simulink model "untitled1"  (R2022a)
settings: Solver=FixedStepDiscrete  StartTime=0.0  StopTime=0.2  FixedStep=0.001  RelTol=1e-3
settings Model: Creator=Administrator  LastModifiedBy=Administrator

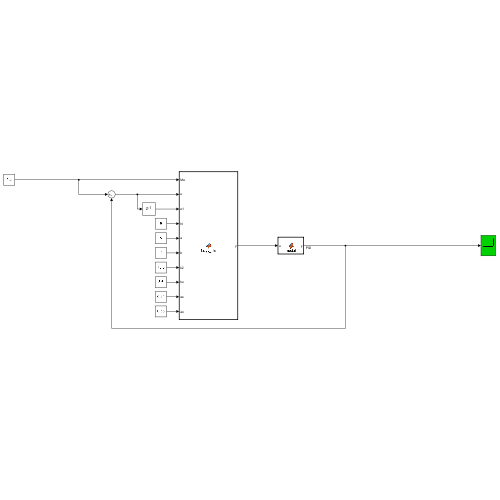
[thumbnail: Simulink's stored preview of the top-level diagram]
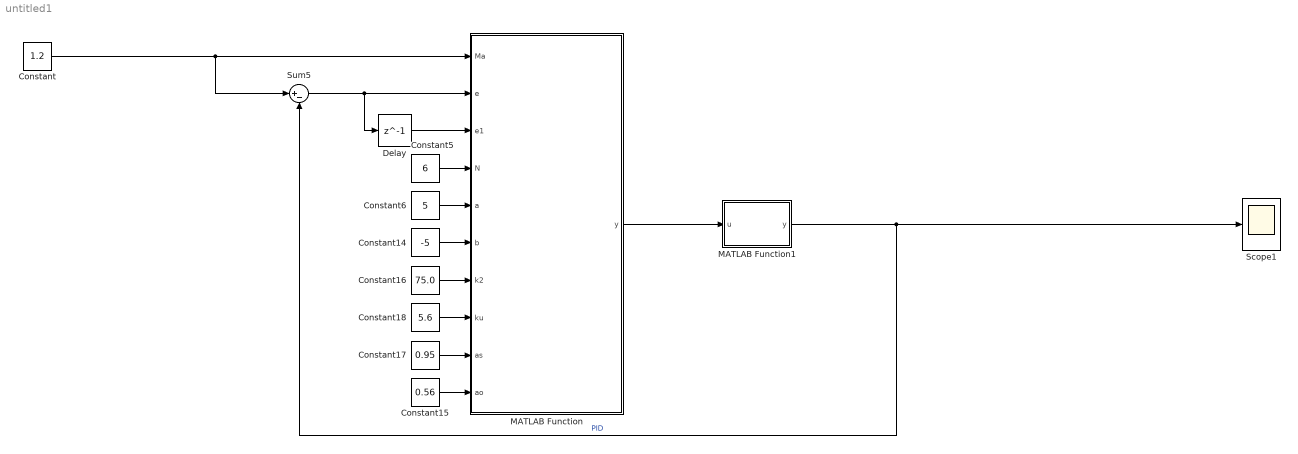
== system untitled1 ==
  Constant : Constant  Value=1.2
  Constant14 : Constant  Value=-5  OutDataTypeStr=Inherit: Inherit via back propagation
  Constant15 : Constant  Value=0.56  OutDataTypeStr=Inherit: Inherit via back propagation
  Constant16 : Constant  Value=75.0  OutDataTypeStr=Inherit: Inherit via back propagation
  Constant17 : Constant  Value=0.95  OutDataTypeStr=Inherit: Inherit via back propagation
  Constant18 : Constant  Value=5.6  OutDataTypeStr=Inherit: Inherit via back propagation
  Constant5 : Constant  Value=6  OutDataTypeStr=Inherit: Inherit via back propagation
  Constant6 : Constant  Value=5
  Delay : Delay  DelayLength=1
  MATLAB Function : MATLAB Function  TreatAsAtomicUnit=on
      settings: MinAlgLoopOccurrences=on
  MATLAB Function1 : MATLAB Function  TreatAsAtomicUnit=on
  Scope1 : Scope
  Sum5 : Sum  Inputs=|+-
  wires:
  Constant6/1 -> MATLAB Function/5(a)
  Constant18/1 -> MATLAB Function/8(ku)
  Constant15/1 -> MATLAB Function/10(ao)
  Sum5/1 -> Delay/1, MATLAB Function/2(e)
  Constant5/1 -> MATLAB Function/4(N)
  Constant14/1 -> MATLAB Function/6(b)
  Constant16/1 -> MATLAB Function/7(k2)
  Constant17/1 -> MATLAB Function/9(as)
  Constant/1 -> MATLAB Function/1(Ma), Sum5/1
  Delay/1 -> MATLAB Function/3(e1)
  MATLAB Function1/1(y) -> Sum5/2, Scope1/1  "PID"
  MATLAB Function/1(y) -> MATLAB Function1/1(u)

== matlab function untitled1/MATLAB Function1 ==
  data: u input; y output
function y = model(u)

y1 = (50)/(14.52*u*u+12.32*u+1);

y = y1;

end

== matlab function untitled1/MATLAB Function ==
  data: Ma input; e input; e1 input; N input; y output; a input; b input; k2 input; ku input; as input; ao input
function y = fuzyy_pid(Ma,e,e1,N,a,b,k2,ku,as,ao)


	ed = e - e1;
	E = -(2 * N) * (e * k2 - (a + b)) / (b - a);    
	E1 = E;
	EC = -(2 * N) * (ed - (a + b)) / (b - a);
	EC1 = 270 * EC;
	a1 = (1 / N) * (as - ao) * abs(E1) + ao;
	y1 = (-(a1 * E1 + (1 - a1) * EC1) / 2);
    y2=y1*ku;
    y=y2*Ma;
    
end
